simulink model "GCS_Fixed_Wing"  (R2025a)
settings: Solver=VariableStepAuto  StartTime=0.0  StopTime=inf  RelTol=1e-3
(part 1 of 2)
settings Model: Creator=gurt1  LastModifiedBy=17036

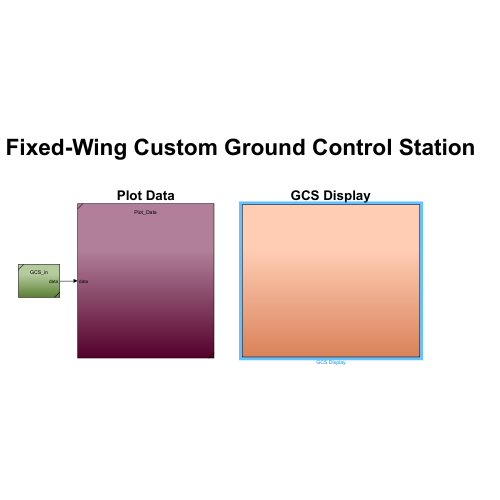
[thumbnail: Simulink's stored preview of the top-level diagram]
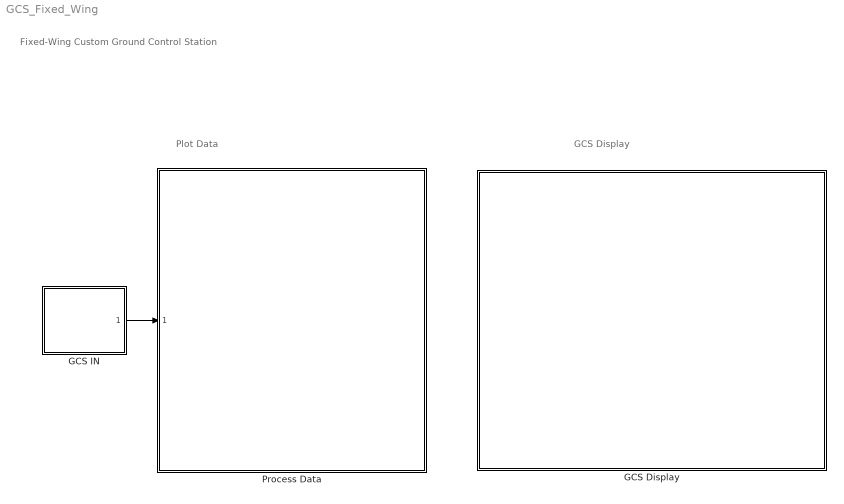
== system GCS_Fixed_Wing ==
  note: Plot Data
  note: GCS Display
  note: Fixed-Wing Custom Ground Control Station
  GCS Display : Subsystem
  GCS IN : Subsystem  ReferencedSubsystem=GCS_in
  Process Data : Subsystem  ReferencedSubsystem=Plot_Data
  wires:
  GCS IN/1 -> Process Data/1
